simulink model "RL_ML_controller"  (R2024b)
settings: Solver=ode1  StartTime=0.0  StopTime=10.0  FixedStep=Ts  RelTol=1e-3
PostLoadFcn:
  | if any(exist('dsrtsu_mdlpostloadfcn', 'file') ~= 0), dsrtsu_mdlpostloadfcn('Execute', bdroot); end
InitFcn:
  | , if any(exist('rtifpga_mdlclblib', 'file') ~= 0), rtifpga_mdlclblib('Init', bdroot); end,
values from neighbouring files (symbols this model uses):
  A = [-45.9636925454  0  4.6929058838; 0  0  1; -28.3611889196  1648.7394958  0]    [controller.mat]    (also in controller_parameters_STUDENT.m = [-R/L0, 0, (Ld*cL*I0)/(L0*((cL+Y0)^2)))
  B = [9.19273850908 0 0]    [controller.mat]
  C = [0 1 0]    [controller.mat]    (also in controller_parameters_STUDENT.m = [0,1,0])
  disable_PWM = 0    [controller.mat]    (also in controller_parameters_STUDENT.m)
  I0 = 0.69179046251    [controller.mat]    (also in controller_parameters_STUDENT.m = sqrt((2*g*m)/(Ld*cL))*(cL+Y0))
  I_Offset_cor = 0    [controller.mat]    (also in controller_parameters_STUDENT.m)
  K = [200.597058824 -300540.891418 -3702.54209359]    [controller.mat]    (also in controller_parameters_STUDENT.m = K_(2:4))
  Ki = -5523230.30591    [controller.mat]    (also in controller_parameters_STUDENT.m = K_(1))
  L = [-274324.956658 1254.03630745 263875.503829]    [controller.mat]    (also in controller_parameters_STUDENT.m = place(A', C', observer_poles)')
  M = 0    [controller.mat]    (also in controller_parameters_STUDENT.m)
  N = 0    [controller.mat]    (also in controller_parameters_STUDENT.m)
  terminate = 0    [controller.mat]    (also in controller_parameters_STUDENT.m)
  Tslf = 0.0002    [controller.mat]    (also in controller_parameters_STUDENT.m)
  U0 = 3.45895231255    [controller.mat]    (also in controller_parameters_STUDENT.m = R*I0)
  x0 = [0.69179046251 0.01 0]    [controller.mat]    (also in controller_parameters_STUDENT.m = [I0,Y0,Ydot0].')
  Y0 = 0.01    [controller.mat]    (also in controller_parameters_STUDENT.m)
libraries: simulink x1
settings Model: DSRTSU_INTERNAL_RTI_VER=560  DSRTSU_INTERNAL_RTI_TYPE=rti1104  RTICANMMDATA=struct('GeneralSetupData',struct('modelroot','E:\RemoteLabs\Teacher_files','generalsettings',struct('filesettings',struct('destfolder',struct('Name','RTICANMM_FILES','Check',1),'buildfolder',struct('Name','.','Check',1),'AbsDestfolder',struct('Name','E:\RemoteLabs\Teacher_files\RTICANMM_FILES'),'AbsBuildfolder',struct('Name','E:\RemoteLabs\Teacher_files'))),'options',struct('addpaths',1,'rmpaths',1,'addtrcexclusion',true,'cannavigator',struct('checkmonitoring',0),'show_usrtrc',0,'use_usrtrc',0),'advanced',struct('options',ones(1,100)),'MPSetup',{{}},'RTI',struct('Type','RTI1104','Ver','7.14','Date','02-May-2020'),'modelname','controller_WL','block','controller_WL'))  DSRTSU_INTERNAL_RTIFPGA=160  Creator=20201603  LastModifiedBy=danieltyukov
settings SolverCC: AlgebraicLoopSolver=TrustRegion
settings OptimizationCC: BlockReduction=off
settings DebuggingCC: UnconnectedInputMsg=warning  UnconnectedOutputMsg=warning  UnconnectedLineMsg=warning
settings HardwareCC: ProdBitPerPointer=32  ProdBitPerSizeT=32  ProdBitPerPtrDiffT=32  ProdLargestAtomicInteger=Integer  ProdEndianess=BigEndian  ProdWordSize=32  ProdHWDeviceType=Custom Processor->Custom  TargetIntDivRoundTo=Zero  TargetEndianess=BigEndian  TargetHWDeviceType=Custom Processor->Custom
settings ModelReferenceCC: EnableRefExpFcnMdlSchedulingChecks=on  ModelReferenceNumInstancesAllowed=Single  ModelReferenceMinAlgLoopOccurrences=on
settings SFSimCC: MATLABDynamicMemAlloc=off
settings RTWCC: Description=dSPACE DS1104 Hardware Platform  SystemTargetFile=rti1104.tlc  MakeCommand=make_rti  TemplateMakefile=rti1104.tmf  GPUComputeCapability=3.5
settings STFCustomTargetCC: ParMdlRefBuildCompliant=on  SystemTargetFile=rti1104.tlc
settings GRTTargetCC: TargetLangStandard=C89/C90 (ANSI)  CompOptLevelCompliant=off  ConcurrentExecutionCompliant=off  CombineOutputUpdateFcns=off  MatFileLogging=off  CPPClassGenCompliant=off  UseToolchainInfoCompliant=off

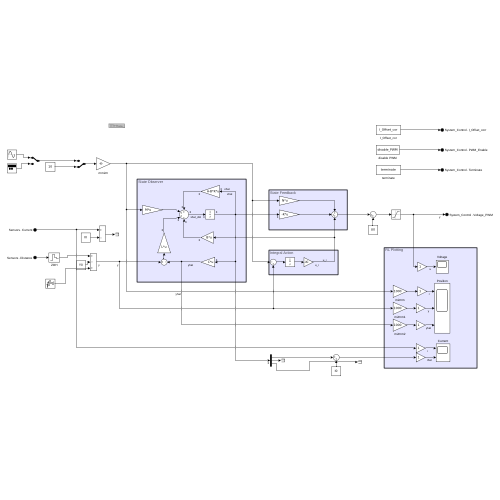
[thumbnail: Simulink's stored preview of the top-level diagram]
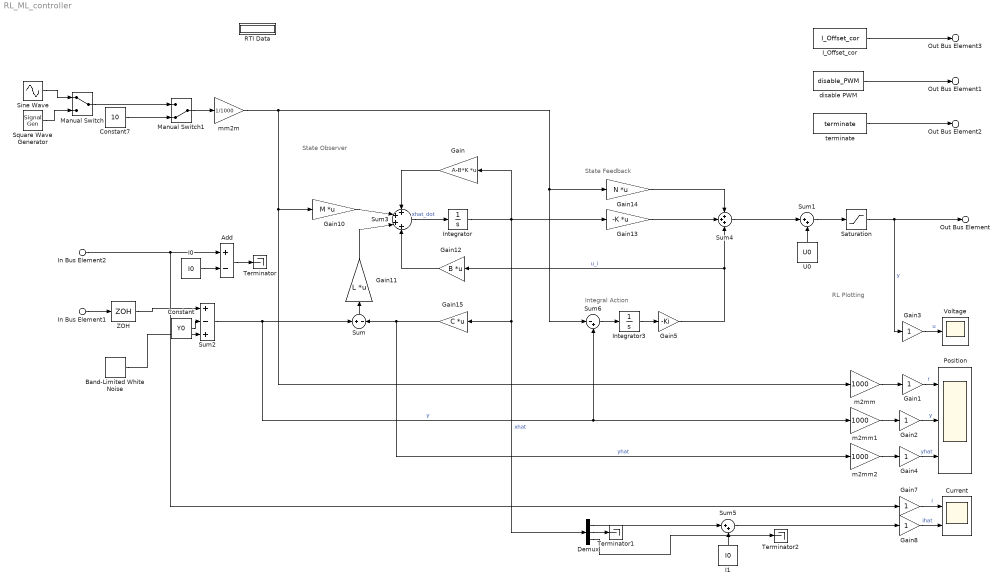
== system RL_ML_controller ==
  note: RL Plotting
  note: Integral Action
  note: State Feedback
  note: State Observer
  In Bus Element1 : Inport  PortName=Sensors  Element=Distance
  In Bus Element2 : Inport  PortName=Sensors  Element=Current
  Add : Sum  Inputs=+-
  Band-Limited White Noise : simulink/Sources/Band-Limited White Noise  Cov=[4e-11]  Ts=0.1  seed=[23341]
  Constant : Constant  Value=Y0
  Constant7 : Constant  Value=10
  Current : Scope  NumInputPorts=2
  Demux : Demux  Outputs=3
  Gain : Gain  Gain=A-B*K  Multiplication=Matrix(K*u)
  Gain{1..4,7..8} (6 alike) : Gain
  Gain10 : Gain  Gain=M  Multiplication=Matrix(K*u)
  Gain11 : Gain  Gain=L  Multiplication=Matrix(K*u)
  Gain12 : Gain  Gain=B  Multiplication=Matrix(K*u)
  Gain13 : Gain  Gain=-K  Multiplication=Matrix(K*u)
  Gain14 : Gain  Gain=N  Multiplication=Matrix(K*u)
  Gain15 : Gain  Gain=C  Multiplication=Matrix(K*u)
  Gain5 : Gain  Gain=-Ki
  I0 : Constant  Value=I0
  I1 : Constant  Value=I0
  I_Offset_cor : Constant  Value=I_Offset_cor  OutDataTypeStr=double
  Integrator : Integrator  InitialCondition=x0
  Integrator3 : Integrator  UpperSaturationLimit=1e-5  LowerSaturationLimit=-1e-5
  Manual Switch : ManualSwitch
  Manual Switch1 : ManualSwitch  CurrentSetting=0
  Position : Scope  NumInputPorts=3
  RTI Data : Subsystem  Tag=struct('RTIDataServer',struct('RTIDataServerVs','2','RTIModelDescription','struct(''main'',''controller_WL'',''sub'','''',''isMp'',0)'))  LoadFcn="if exist('rtidc'), try,  rtidc('DataHostBlockClbLoad', gcbh); catch, disp(['Warning: ''LoadFcn'' for RTI Data block failed: ' lasterr]); end, end,"  mask(RTI_DATA_HOST){}
      mask help:
      | RTI Data Block.
      | This block is used by RTI to store internal model-dependent data.
      | Please keep this block on the root level of the model. Deleting this block will result in data loss.
      |
      | NEVER DELETE OR COPY THIS BLOCK!
      settings: CopyFcn="if exist('rtidc'), try,  rtidc('DataHostBlockClbCopy', gcbh); catch, disp(['Warning: ''CopyFcn'' for RTI Data block failed: ' lasterr]); end, end,"  DeleteFcn="if exist('rtidc'), try,  rtidc('DataHostBlockClbDelete', gcbh); catch, disp(['Warning: ''DeleteFcn'' for RTI Data block failed: ' lasterr]); end, end,"  ModelCloseFcn="if exist('rtidc'), try,  rtidc('DataHostBlockClbModelClose', gcbh); catch, disp(['Warning: ''ModelCloseFcn'' for RTI Data block failed: ' lasterr]); end, end,"  PreSaveFcn="if exist('rtidc'), try,  rtidc('DataHostBlockClbPreSave', gcbh); catch, disp(['Warning: ''PreSaveFcn'' for RTI Data block failed: ' lasterr]); end, end,"  PostSaveFcn="if exist('rtidc'), try,  rtidc('DataHostBlockClbPostSave', gcbh); catch, disp(['Warning: ''PostSaveFcn'' for RTI Data block failed: ' lasterr]); end, end,"  NameChangeFcn="if exist('rtidc'), try,  rtidc('DataHostBlockClbNameChange', gcbh); catch, disp(['Warning: ''NameChangeFcn'' for RTI Data block failed: ' lasterr]); end, end,"
      mask Help:
      | RTI Data Block.
      | This block is used by RTI to store internal model-dependent data.
      | Please keep this block on the root level of the model. Deleting this block will result in data loss.
      | 
      | NEVER DELETE OR COPY THIS BLOCK!
      mask Display:
      | text(0.5, 0.5, 'RTI Data', 'HorizontalAlignment', 'center');
      | plot([1 0]);
  Saturation : Saturate  UpperLimit=12  LowerLimit=0
  Sine Wave : Sin  Frequency=2*pi  SampleTime=0
  Square Wave Generator : SignalGenerator  WaveForm=square  Amplitude=0.5  Frequency=0.5
  Sum : Sum  Inputs=+|-
  Sum1 : Sum  Inputs=|++
  Sum2 : Sum  Inputs=+-+
  Sum3 : Sum  Inputs=++++
  Sum4 : Sum  Inputs=+++
  Sum5 : Sum  Inputs=|++
  Sum6 : Sum  Inputs=|-+
  Terminator : Terminator
  Terminator1 : Terminator
  Terminator2 : Terminator
  U0 : Constant  Value=U0
  Voltage : Scope
  ZOH : ZeroOrderHold  SampleTime=Tslf
  disable PWM : Constant  Value=disable_PWM  OutDataTypeStr=double
  m2mm : Gain  Gain=1000
  m2mm1 : Gain  Gain=1000
  m2mm2 : Gain  Gain=1000
  mm2m : Gain  Gain=1/1000
  terminate : Constant  Value=terminate  OutDataTypeStr=double
  Out Bus Element : Outport  PortName=System_Control  Element=Voltage_PWM
  Out Bus Element1 : Outport  PortName=System_Control  Element=PWM_Enable
  Out Bus Element2 : Outport  PortName=System_Control  Element=Terminate
  Out Bus Element3 : Outport  PortName=System_Control  Element=I_Offset_corr
  wires:
  Constant/1 -> Sum2/2
  U0/1 -> Sum1/2
  I0/1 -> Add/2
  terminate/1 -> Out Bus Element2/1
  disable PWM/1 -> Out Bus Element1/1
  I_Offset_cor/1 -> Out Bus Element3/1
  Gain1/1 -> Position/1  "r"
  m2mm/1 -> Gain1/1
  Gain2/1 -> Position/2  "y"
  Gain3/1 -> Voltage/1  "u"
  Sum2/1 -> m2mm1/1, Sum6/2, Sum/1  "y"
  In Bus Element2/1 -> Add/1, Gain7/1
  Sum/1 -> Gain11/1
  Integrator/1 -> Gain13/1, Demux/1, Gain15/1, Gain/1  "xhat"
  Gain/1 -> Sum3/1
  Gain15/1 -> m2mm2/1, Sum/2  "yhat"
  Gain11/1 -> Sum3/3
  Gain10/1 -> Sum3/2
  Gain13/1 -> Sum4/2
  Gain14/1 -> Sum4/1
  Sum4/1 -> Sum1/1
  Add/1 -> Terminator/1
  mm2m/1 -> Sum6/1, Gain14/1, m2mm/1, Gain10/1
  m2mm1/1 -> Gain2/1
  Sine Wave/1 -> Manual Switch/1
  Square Wave Generator/1 -> Manual Switch/2
  Integrator3/1 -> Gain5/1
  Gain5/1 -> Sum4/3, Gain12/1  "u_i"
  m2mm2/1 -> Gain4/1
  Gain4/1 -> Position/3  "yhat"
  Gain7/1 -> Current/1  "i"
  Manual Switch/1 -> Manual Switch1/1
  Manual Switch1/1 -> mm2m/1
  Sum1/1 -> Saturation/1
  Gain8/1 -> Current/2  "ihat"
  Sum5/1 -> Gain8/1
  I1/1 -> Sum5/2
  ZOH/1 -> Sum2/1
  Sum6/1 -> Integrator3/1
  Saturation/1 -> Out Bus Element/1, Gain3/1  "y"
  In Bus Element1/1 -> ZOH/1
  Sum3/1 -> Integrator/1  "xhat_dot"
  Gain12/1 -> Sum3/4
  Demux/1 -> Sum5/1
  Demux/2 -> Terminator1/1
  Demux/3 -> Terminator2/1
  Constant7/1 -> Manual Switch1/2
  Band-Limited White Noise/1 -> Sum2/3

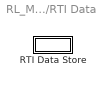
== system RL_ML_controller/RTI Data ==
  RTI Data Store : Subsystem  Tag="struct('private',struct('version',struct('dsVer',uint32(2),'dsVerCreation',uint32(2),'RTI',struct('ver','7.14','type','RTI1104')),'access',struct('type','Model','isPerm',1,'created',['27-Jul-2020 15:03:57'],'modified',['31-Jul-2020 11:34:33'],'location','')),'public',struct('main',struct('data',[]),'sub',struct('name',{{'controller_WL'}},'data',{{struct('TH',struct('thTaskInfo',struct('taskType',{'TIMER','HWINT','TMRINT','SWINT','GLINT'},'tasksNumOf',{1,0,0,0,0},'srcIds',{{'TIMERA'},{},{},{},{}},'taskNames',{{['Timer Task 1']},{},{},{},{}})),'th_tc',struct('dataType','TASK','taskGroupId','','taskGroupList',{{}},'taskSchedulingPolicy','FCFS','taskType','TIMER','blkh',-1,'srcId','TIMERA','srcSgnName',['Timer A interrupt'],'srcCpuName','','taskName',['Timer Task 1  [0.0002] s'],'taskNameDisplayExt','','smplTime',0.0002,'smplTimeOffs',0,'hasFixedPriority',0,'priority',1,'hasFixedOvc',0,'ovcType',1,'ovcMax',1),'tc_th',struct('dataType','TASK','taskGroupId','','taskGroupList',{{}},'taskSchedulingPolicy','FCFS','taskType','TIMER','blkh',-1,'srcId','TIMERA','srcSgnName',['Timer A interrupt'],'srcCpuName','','taskName',['Timer Task 1  [0.0002] s'],'taskNameDisplayExt','','smplTime',0.0002,'smplTimeOffs',0,'hasFixedPriority',0,'priority',1,'hasFixedOvc',0,'ovcType',1,'ovcMax',1))}})))"  mask(RTI_DATA_STORE){}
      mask help:
      | RTI Data Store Block. This block is used by RTI to store internal model dependent data. Deleting this block will result in data loss.
      |
      | NEVER DELETE, COPY, OR MODIFY THIS BLOCK!
      mask Help:
      | RTI Data Store Block. This block is used by RTI to store internal model dependent data. Deleting this block will result in data loss.
      | 
      | NEVER DELETE, COPY, OR MODIFY THIS BLOCK!
      mask Display: text(0.5, 0.5, ' ', 'HorizontalAlignment', 'center');

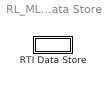
== system RL_ML_controller/RTI Data/RTI Data Store ==
  RTI Data Store : Subsystem  mask(RTI_DATA_STORE){}
      mask help:
      | RTI Data Store Block. This block is used by RTI to store internal model dependent data. Deleting this block will result in data loss.
      |
      | NEVER DELETE, COPY, OR MODIFY THIS BLOCK!
      mask Help:
      | RTI Data Store Block. This block is used by RTI to store internal model dependent data. Deleting this block will result in data loss.
      | 
      | NEVER DELETE, COPY, OR MODIFY THIS BLOCK!
      mask Display: text(0.5, 0.5, ' ', 'HorizontalAlignment', 'center');

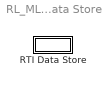
== system RL_ML_controller/RTI Data/RTI Data Store/RTI Data Store ==
  RTI Data Store : Subsystem  mask(RTI_DATA_STORE){}
      mask help:
      | RTI Data Store Block. This block is used by RTI to store internal model dependent data. Deleting this block will result in data loss.
      |
      | NEVER DELETE, COPY, OR MODIFY THIS BLOCK!
      mask Help:
      | RTI Data Store Block. This block is used by RTI to store internal model dependent data. Deleting this block will result in data loss.
      | 
      | NEVER DELETE, COPY, OR MODIFY THIS BLOCK!
      mask Display: text(0.5, 0.5, ' ', 'HorizontalAlignment', 'center');

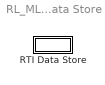
== system RL_ML_controller/RTI Data/RTI Data Store/RTI Data Store/RTI Data Store ==
  RTI Data Store : Subsystem  mask(RTI_DATA_STORE){}
      mask help:
      | RTI Data Store Block. This block is used by RTI to store internal model dependent data. Deleting this block will result in data loss.
      |
      | NEVER DELETE, COPY, OR MODIFY THIS BLOCK!
      mask Help:
      | RTI Data Store Block. This block is used by RTI to store internal model dependent data. Deleting this block will result in data loss.
      | 
      | NEVER DELETE, COPY, OR MODIFY THIS BLOCK!
      mask Display: text(0.5, 0.5, ' ', 'HorizontalAlignment', 'center');

== system RL_ML_controller/RTI Data/RTI Data Store/RTI Data Store/RTI Data Store/RTI Data Store ==
